simulink model "SYSTEM"  (R2019b)
settings: Solver=VariableStepAuto  StartTime=0.0  StopTime=10.0  RelTol=1e-3
values from neighbouring files (symbols this model uses):
  Dactl = Dactr    [WEIGHTS.m]
  Dactr = zpk([],[-0.2],0.15)    [WEIGHTS.m]
  Wg = zpk([],[],0.01)    [WEIGHTS.m]
  Wn = zpk([-0.1],[-100], 100)    [WEIGHTS.m]
  Wt = zpk([],[-3e-3],0.04)    [WEIGHTS.m]
  Wtaul = Wtaur    [WEIGHTS.m]
  Wtaur = zpk([-1],[-1000],6)    [WEIGHTS.m]
  Wu = zpk([],[-1e-2],0.1)    [WEIGHTS.m]
undefined symbols (not defined in the file or in its folder): segway
settings Model: Creator=Abolfazl  LastModifiedBy=Abolfazl

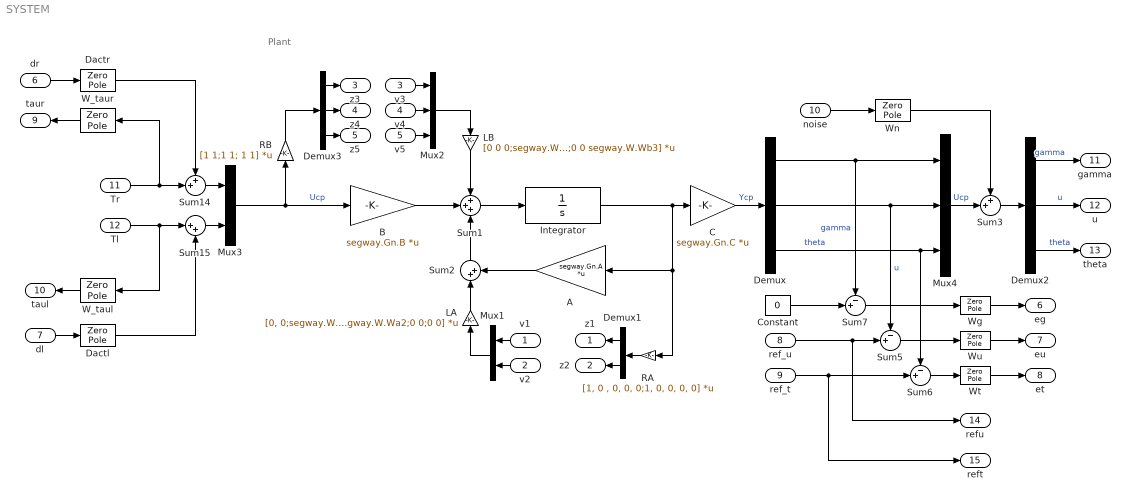
== system SYSTEM ==
  note: Plant
  v1 : Inport
  v2 : Inport  Port=2
  v3 : Inport  Port=3
  v4 : Inport  Port=4
  v5 : Inport  Port=5
  dr : Inport  Port=6
  dl : Inport  Port=7
  ref_u : Inport  Port=8
  ref_t : Inport  Port=9
  noise : Inport  Port=10
  Tr : Inport  Port=11
  Tl : Inport  Port=12
  A : Gain  Gain=segway.Gn.A  Multiplication=Matrix(K*u)
  B : Gain  Gain=segway.Gn.B  Multiplication=Matrix(K*u)
  C : Gain  Gain=segway.Gn.C  Multiplication=Matrix(K*u)
  Constant : Constant  Value=0
  Dactl : ZeroPole  Zeros=Dactl.Z{:}  Poles=Dactl.P{:}  Gain=Dactl.K
  Dactr : ZeroPole  Zeros=Dactr.Z{:}  Poles=Dactr.P{:}  Gain=Dactr.K
  Demux : Demux  Outputs=3
  Demux1 : Demux  Outputs=2
  Demux2 : Demux  Outputs=3
  Demux3 : Demux  Outputs=3
  Integrator : Integrator
  LA : Gain  Gain=[0, 0;segway.W.Wa1 0;0 segway.W.Wa2;0 0;0 0]  Multiplication=Matrix(K*u)
  LB : Gain  Gain=[0 0 0;segway.W.Wb1 0 0;0 segway.W.Wb2 0;0 0 0;0 0 segway.W.Wb3]  Multiplication=Matrix(K*u)
  Mux1 : Mux  Inputs=2
  Mux2 : Mux  Inputs=3
  Mux3 : Mux  Inputs=2
  Mux4 : Mux  Inputs=3
  RA : Gain  Gain=[1, 0 , 0, 0, 0;1, 0, 0, 0, 0]  Multiplication=Matrix(K*u)
  RB : Gain  Gain=[1 1;1 1; 1 1]  Multiplication=Matrix(K*u)
  Sum1 : Sum  Inputs=+++
  Sum14 : Sum  Inputs=++|
  Sum15 : Sum  Inputs=|++
  Sum2 : Sum  Inputs=|++
  Sum3 : Sum  Inputs=++|
  Sum5 : Sum  Inputs=-+|
  Sum6 : Sum  Inputs=-+|
  Sum7 : Sum  Inputs=-+|
  W_taul : ZeroPole  Zeros=Wtaul.Z{:}  Poles=Wtaul.P{:}  Gain=Wtaul.K
  W_taur : ZeroPole  Zeros=Wtaur.Z{:}  Poles=Wtaur.P{:}  Gain=Wtaur.K
  Wg : ZeroPole  Zeros=Wg.Z{:}  Poles=Wg.P{:}  Gain=Wg.K
  Wn : ZeroPole  Zeros=Wn.Z{:}  Poles=Wn.P{:}  Gain=Wn.K
  Wt : ZeroPole  Zeros=Wt.Z{:}  Poles=Wt.P{:}  Gain=Wt.K
  Wu : ZeroPole  Zeros=Wu.Z{:}  Poles=Wu.P{:}  Gain=Wu.K
  z1 : Outport
  z2 : Outport  Port=2
  z3 : Outport  Port=3
  z4 : Outport  Port=4
  z5 : Outport  Port=5
  eg : Outport  Port=6
  eu : Outport  Port=7
  et : Outport  Port=8
  taur : Outport  Port=9
  taul : Outport  Port=10
  gamma : Outport  Port=11
  u : Outport  Port=12
  theta : Outport  Port=13
  refu : Outport  Port=14
  reft : Outport  Port=15
  wires:
  dr/1 -> Dactr/1
  dl/1 -> Dactl/1
  ref_u/1 -> refu/1, Sum5/2
  ref_t/1 -> reft/1, Sum6/2
  Constant/1 -> Sum7/2
  Wg/1 -> eg/1
  Sum7/1 -> Wg/1
  Wu/1 -> eu/1
  Sum5/1 -> Wu/1
  Wt/1 -> et/1
  Sum6/1 -> Wt/1
  W_taur/1 -> taur/1
  W_taul/1 -> taul/1
  Sum14/1 -> Mux3/1
  Sum15/1 -> Mux3/2
  Dactr/1 -> Sum14/1
  Dactl/1 -> Sum15/2
  Tl/1 -> Sum15/1, W_taul/1
  Tr/1 -> Sum14/2, W_taur/1
  noise/1 -> Wn/1
  Sum1/1 -> Integrator/1
  B/1 -> Sum1/2
  Mux3/1 -> RB/1, B/1  "Ucp"
  A/1 -> Sum2/2
  Sum2/1 -> Sum1/3
  Integrator/1 -> C/1, A/1, RA/1
  Wn/1 -> Sum3/1
  Demux1/1 -> z1/1
  Demux1/2 -> z2/1
  v1/1 -> Mux1/1
  v2/1 -> Mux1/2
  Demux3/2 -> z4/1
  Demux3/1 -> z3/1
  v4/1 -> Mux2/2
  v3/1 -> Mux2/1
  Demux3/3 -> z5/1
  v5/1 -> Mux2/3
  Demux/1 -> Mux4/1, Sum7/1  "gamma"
  Demux/2 -> Mux4/2, Sum5/1  "u"
  Demux/3 -> Mux4/3, Sum6/1  "theta"
  Mux2/1 -> LB/1
  LB/1 -> Sum1/1
  RB/1 -> Demux3/1
  RA/1 -> Demux1/1
  LA/1 -> Sum2/1
  Mux1/1 -> LA/1
  C/1 -> Demux/1  "Ycp"
  Demux2/1 -> gamma/1  "gamma"
  Demux2/2 -> u/1  "u"
  Demux2/3 -> theta/1  "theta"
  Sum3/1 -> Demux2/1
  Mux4/1 -> Sum3/2  "Ucp"
